simulink model "without_ff"  (R2018a)
settings: Solver=VariableStepAuto  StartTime=0.0  StopTime=30  RelTol=1e-3
settings Model: Creator=Halil Temurtaş  LastModifiedBy=Halil Temurtaş

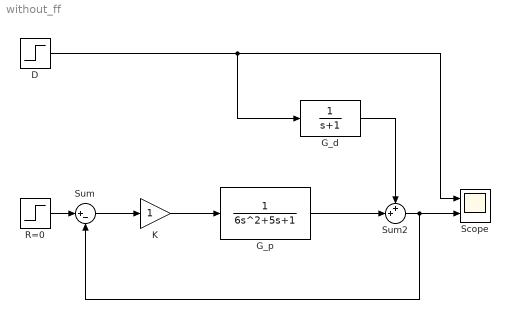
== system without_ff ==
  D : Step  SampleTime=0
  G_d : TransferFcn  Denominator=[1 1]
  G_p : TransferFcn  Denominator=[6 5 1]
  K : Gain
  "R=0 " : Step  After=0  SampleTime=0
  Scope : Scope  NumInputPorts=2
  Sum : Sum  Inputs=|+-
  Sum2 : Sum  Inputs=++|
  wires:
  "R=0 "/1 -> Sum/1
  Sum/1 -> K/1
  K/1 -> G_p/1
  G_p/1 -> Sum2/2
  G_d/1 -> Sum2/1
  D/1 -> Scope/1, G_d/1
  Sum2/1 -> Sum/2, Scope/2
